simulink model "GananciaProgramadaSim"  (R2022b)
settings: Solver=ode45  StartTime=0.0  StopTime=600  RelTol=1e-3
values from neighbouring files (symbols this model uses):
  q0coe = polyfit(u,q0,4)    [GananciaProgramadaLab2.m]
  q1coe = polyfit(u,q1,4)    [GananciaProgramadaLab2.m]
  q2coe = polyfit(u,q2,4)    [GananciaProgramadaLab2.m]
  T = 0.001    [GananciaProgramadaLab2.m]    (also in MRACdiscretoLab2.m = 0.470737468013)
undefined symbols (not defined in the file or in its folder): dt, nt, retardos
libraries: simulink x1
settings Model: Creator=salas  LastModifiedBy=emanu
settings ModelReferenceCC: EnableRefExpFcnMdlSchedulingChecks=on

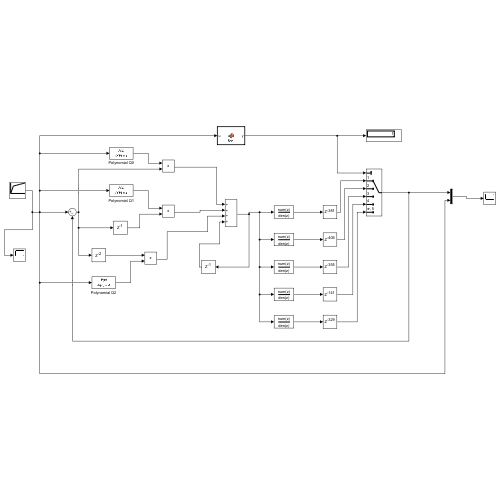
[thumbnail: Simulink's stored preview of the top-level diagram]
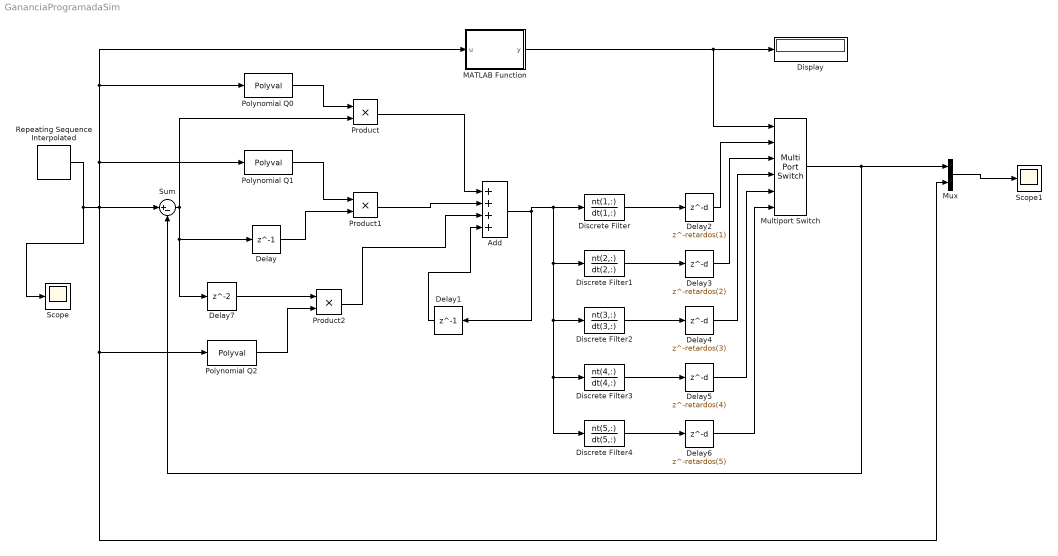
== system GananciaProgramadaSim ==
  Add : Sum  Inputs=++++
  Delay : Delay  DelayLength=1  SampleTime=T
  Delay1 : Delay  DelayLength=1  SampleTime=T
  Delay2 : Delay  DelayLength=retardos(1)  SampleTime=T
  Delay3 : Delay  DelayLength=retardos(2)  SampleTime=T
  Delay4 : Delay  DelayLength=retardos(3)  SampleTime=T
  Delay5 : Delay  DelayLength=retardos(4)  SampleTime=T
  Delay6 : Delay  DelayLength=retardos(5)  SampleTime=T
  Delay7 : Delay  SampleTime=T
  Discrete Filter : DiscreteFilter  Numerator=nt(1,:)  Denominator=dt(1,:)  SampleTime=T
  Discrete Filter1 : DiscreteFilter  Numerator=nt(2,:)  Denominator=dt(2,:)  SampleTime=T
  Discrete Filter2 : DiscreteFilter  Numerator=nt(3,:)  Denominator=dt(3,:)  SampleTime=T
  Discrete Filter3 : DiscreteFilter  Numerator=nt(4,:)  Denominator=dt(4,:)  SampleTime=T
  Discrete Filter4 : DiscreteFilter  Numerator=nt(5,:)  Denominator=dt(5,:)  SampleTime=T
  Display : Display
  MATLAB Function : MATLAB Function  TreatAsAtomicUnit=on
  Multiport Switch : MultiPortSwitch  Inputs=5  SaturateOnIntegerOverflow=off  InputSameDT=off
  Mux : Mux  Inputs=2
  Polynomial Q0 : Polyval  Coefs=q0coe
  Polynomial Q1 : Polyval  Coefs=q1coe
  Polynomial Q2 : Polyval  Coefs=q2coe
  Product : Product
  Product1 : Product
  Product2 : Product
  Repeating Sequence Interpolated : simulink/Sources/Repeating Sequence Interpolated  OutValues=[0 38 42 46 50 54]  TimeValues=[0 100 200 300 400 500]  LookUpMeth=Interpolation-Use End Values  tsamp=100  OutMin=[]  OutMax=[]  OutDataTypeStr=double  OutputDataTypeScalingMode=double  OutDataType=fixdt(0,8)  OutScaling=2^-10
  Scope : Scope
  Scope1 : Scope
  Sum : Sum  Inputs=|+-
  wires:
  Sum/1 -> Delay7/1, Delay/1, Product/2
  Polynomial Q0/1 -> Product/1
  Add/1 -> Discrete Filter/1, Discrete Filter1/1, Discrete Filter2/1, Discrete Filter4/1, Discrete Filter3/1, Delay1/1
  Product/1 -> Add/1
  Polynomial Q1/1 -> Product1/1
  Delay/1 -> Product1/2
  Product1/1 -> Add/2
  Multiport Switch/1 -> Mux/1, Sum/2
  MATLAB Function/1(y) -> Display/1, Multiport Switch/1
  Discrete Filter4/1 -> Delay6/1
  Discrete Filter3/1 -> Delay5/1
  Discrete Filter2/1 -> Delay4/1
  Discrete Filter1/1 -> Delay3/1
  Discrete Filter/1 -> Delay2/1
  Delay2/1 -> Multiport Switch/2
  Delay3/1 -> Multiport Switch/3
  Delay5/1 -> Multiport Switch/5
  Delay6/1 -> Multiport Switch/6
  Delay1/1 -> Add/4
  Delay7/1 -> Product2/1
  Polynomial Q2/1 -> Product2/2
  Repeating Sequence Interpolated/1 -> Scope/1, Polynomial Q2/1, Mux/2, Polynomial Q1/1, MATLAB Function/1(u), Polynomial Q0/1, Sum/1
  Delay4/1 -> Multiport Switch/4
  Product2/1 -> Add/3
  Mux/1 -> Scope1/1

== matlab function GananciaProgramadaSim/MATLAB Function ==
  data: u input; y output
function y = fcn(u)
y=1;

switch u

    case 38
        y=1;
    case  42 
        y=2;
    case 46
        y=3;
    case 50
        y=4;
    case 54
        y=5;
end
